simulink model "stimulation_one_pair"  (R2023b)
settings: Solver=FixedStepDiscrete  StartTime=0.0  StopTime=inf  RelTol=1e-3  EnableMultiTasking=on
undefined symbols (not defined in the file or in its folder): ES, PULSE, TRAIN
libraries: Tools x1, gEstimPRO x1
settings Model: ModifiedByFormat=g.tec  Creator=nhoyh  LastModifiedBy=g.tec
settings SolverCC: AlgebraicLoopSolver=TrustRegion
settings DataIOCC: LimitDataPoints=on  SaveFormat=Array  ReturnWorkspaceOutputs=off
settings OptimizationCC: LifeSpan=inf
settings DebuggingCC: UnconnectedInputMsg=warning  UnconnectedOutputMsg=warning  UnconnectedLineMsg=warning  SFUnexpectedBacktrackingDiag=warning  SFNoUnconditionalDefaultTransitionDiag=warning  SFExecutionAtInitializationDiag=none  ArithmeticOperatorsInVariantConditions=warning
settings HardwareCC: ProdBitPerPointer=32  ProdBitPerSizeT=32  ProdBitPerPtrDiffT=32  ProdLargestAtomicFloat=None  ProdIntDivRoundTo=Undefined  ProdEndianess=Unspecified  ProdWordSize=32  ProdHWDeviceType=32-bit Generic
settings ModelReferenceCC: EnableRefExpFcnMdlSchedulingChecks=on  PropagateSignalLabelsOutOfModel=off
settings SFSimCC: SimUseLocalCustomCode=off  CustomCodeUndefinedFunction=UseInterfaceOnly
settings RTWCC: RTWUseLocalCustomCode=off
settings CodeAppCC: StateflowObjectComments=on
settings GRTTargetCC: TargetLangStandard=C89/C90 (ANSI)
settings ConfigComp: CovMetricSettings=dw  CovSaveCumulativeToWorkspaceVar=on  CovSaveSingleToWorkspaceVar=on  CovExternalEMLEnable=off

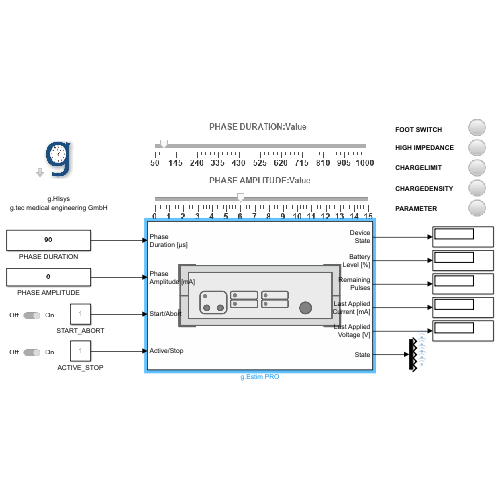
[thumbnail: Simulink's stored preview of the top-level diagram]
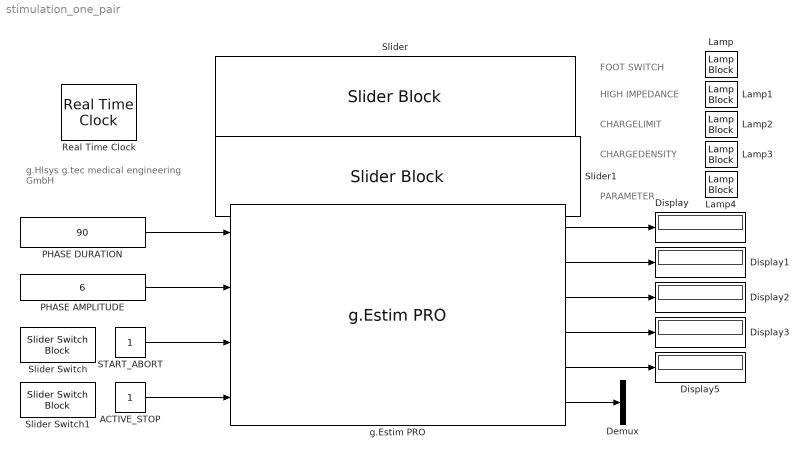
== system stimulation_one_pair ==
  note: g.HIsys
      | g.tec medical engineering GmbH
  note: FOOT SWITCH
  note: HIGH IMPEDANCE
  note: CHARGELIMIT
  note: CHARGEDENSITY
  note: PARAMETER
  ACTIVE_STOP : Constant  SampleTime=0.1
  Demux : Demux  Outputs=5
  Display{,1..3,5} (5 alike) : Display
  Lamp{,1..4} (5 alike) : LampBlock  LabelPosition=Hide
  PHASE AMPLITUDE : Constant  Value=6  SampleTime=0.1
  PHASE DURATION : Constant  Value=90  SampleTime=0.1
  Real Time Clock : Tools/Real Time Clock  timeprofile=off
      settings: SourceProductName=g.HIsys
  START_ABORT : Constant  SampleTime=0.1
  Slider : SliderBlock  ScaleMin=50  ScaleMax=1000
  Slider Switch : SliderSwitchBlock  LabelPosition=Hide
      settings: Values={{'Off', 'On'}, [0 1]}
  Slider Switch1 : SliderSwitchBlock  LabelPosition=Hide
      settings: Values={{'Off', 'On'}, [0 1]}
  Slider1 : SliderBlock  ScaleMax=15
  g.Estim PRO : gEstimPRO/g.Estim PRO  serial=ES-2020.04.02  auto_connect=off  old_serial=ES-2020.04.02  supermode_enabled=off  DI1_enabled=off  buzzer_enabled=on  surface_area_mm2=4.5616  interphase_time=0  modality=BIPHASIC  polarity=ALTERNATING  pulses=19500  pulse_rate=130  fade_type=AMPLITUDE  fade_in_time=0  fade_out_time=0  digout1_mode=2 - PULSE  digout1_pre=1  digout1_post=0  digout2_mode=1 - TRAIN  digout2_pre=2  digout2_post=0
      settings: SourceProductName=g.HIsys
  wires:
  g.Estim PRO/1 -> Display/1
  g.Estim PRO/2 -> Display1/1
  g.Estim PRO/3 -> Display2/1
  g.Estim PRO/5 -> Display5/1
  g.Estim PRO/4 -> Display3/1
  PHASE DURATION/1 -> g.Estim PRO/1
  PHASE AMPLITUDE/1 -> g.Estim PRO/2
  g.Estim PRO/6 -> Demux/1
  ACTIVE_STOP/1 -> g.Estim PRO/4
  START_ABORT/1 -> g.Estim PRO/3
